simulink model "New_vapourcontent"  (Simulink 7.9)
settings: Solver=FixedStepDiscrete  StartTime=0.0  StopTime=10  FixedStep=1  RelTol=1e-3
undefined symbols (not defined in the file): Carnot_vapourcontent_Callbacks
settings Model: Creator=awohlfei  LastModifiedBy=awohlfei

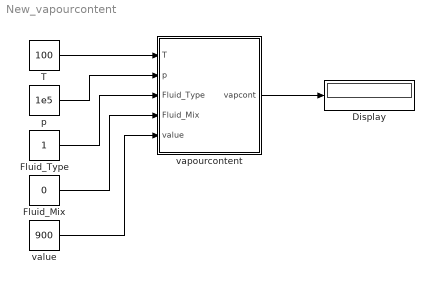
== system New_vapourcontent ==
  Display : Display
  Fluid_Mix : Constant  Value=0
  Fluid_Type : Constant
  T : Constant  Value=100
  p : Constant  Value=1e5
  value : Constant  Value=900
  vapourcontent : Subsystem  LoadFcn=Carnot_vapourcontent_Callbacks('LoadFcn');  InitFcn=load('THB.mat');  VariantObject=CarlibClassic  mask(vapourcontent){INPUTARGUMENTS=state variables (classic), PROPERTYTYPE=density, DEBUGLEVEL=WARNING, MAXTOTALMESSAGES=inf, MAXCONSECUTIVEMESSAGES=inf, WRITETOFILE=0, FILENAME='errors.txt'}
      mask prompts: INPUTARGUMENTS "Input arguments"; PROPERTYTYPE "property type"; DEBUGLEVEL "Debug level"; MAXTOTALMESSAGES "maximum number of total warning"; MAXCONSECUTIVEMESSAGES "maximum number of consecutive warnings"; WRITETOFILE "write messages to file"; FILENAME "filename for error messages"
      mask help:
      | The block calculates the vapour content of fluid [0..1] by the value of a specified property. The block calls the function "vapourcontent" in the CARNOT library "Carlib".
      |
      | Definition of property-types
      | property                    unit
      |  density                     [kg/m³]
      |  heat capacity           [J/kgK]
      |  heat conductivity     [W/mK]
      |  kinematic viscosity   [m²/s]
      |  enthalpy                   [J/kg]
      |  entropy                     [J/kgK]
      |  prandtl                      [-]
      |  specific volume        [m³/kg]
      mask init:
      | %Inports
      | Carnot_vapourcontent_Callbacks('CreateInports');
      | 
      | %global debug level
      | [DEBUGLEVEL, MAXTOTALMESSAGES, MAXCONSECUTIVEMESSAGES, WRITETOFILE, FILENAME] = Carnot_vapourcontent_Callbacks('CheckDebugLevels', DEBUGLEVEL, MAXTOTALMESSAGES, MAXCONSECUTIVEMESSAGES, WRITETOFILE, FILENAME);
      mask Help: eval('man(''vapourcontent'')')
      mask StyleString: popup(state variables (classic)|THB|THV),popup(density|heat capacity|heat conductivity|kinematic viscosity|enthalpy|entropy|prandtl|specific volume),popup(DEBUG|INFO|WARNING|ERROR|FATAL|NONE),edit,edit,edit,edit
      mask CallbackString: Carnot_vapourcontent_Callbacks('MaskVisibilities');||||||
      mask TabNameString: Parameters,Parameters,Debugging,Debugging,Debugging,Debugging,Debugging
  wires:
  vapourcontent/1(vapcont) -> Display/1
  T/1 -> vapourcontent/1(T)
  p/1 -> vapourcontent/2(p)
  Fluid_Type/1 -> vapourcontent/3(Fluid_Type)
  Fluid_Mix/1 -> vapourcontent/4(Fluid_Mix)
  value/1 -> vapourcontent/5(value)

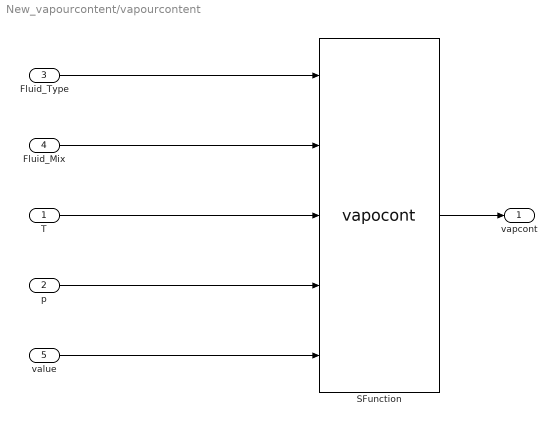
== system New_vapourcontent/vapourcontent ==
  T : Inport
  p : Inport  Port=2
  Fluid_Type : Inport  Port=3
  Fluid_Mix : Inport  Port=4
  value : Inport  Port=5
  SFunction : S-Function  FunctionName=vapocont  Parameters=PROPERTYTYPE, DEBUGLEVEL, MAXTOTALMESSAGES, MAXCONSECUTIVEMESSAGES,WRITETOFILE, FILENAME  EnableBusSupport=off
  vapcont : Outport
  wires:
  SFunction/1 -> vapcont/1
  T/1 -> SFunction/3
  p/1 -> SFunction/4
  Fluid_Type/1 -> SFunction/1
  Fluid_Mix/1 -> SFunction/2
  value/1 -> SFunction/5
